simulink model "control_lazo_cerrado_helicoptero"  (R2015a)
settings: Solver=ode45  StartTime=0.0  StopTime=300  RelTol=1e-3
libraries: arduino_io_lib x8
settings Model: CovHtmlReporting=off  Creator=Alumno  LastModifiedBy=Usuario
settings DataIOCC: LimitDataPoints=off  SaveFormat=Dataset
settings HardwareCC: ProdBitPerPointer=64  ProdLargestAtomicFloat=Float  ProdIntDivRoundTo=Zero  ProdEndianess=LittleEndian  ProdHWDeviceType=Specified
settings ModelReferenceCC: PropagateSignalLabelsOutOfModel=on

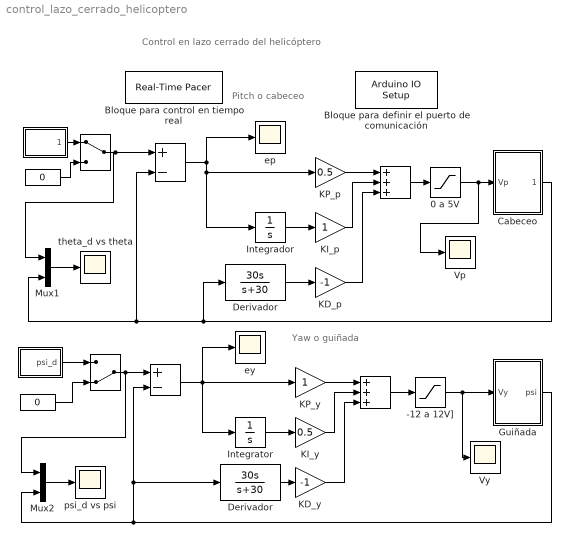
== system control_lazo_cerrado_helicoptero ==
  note: Yaw o guiñada
  note: Pitch o cabeceo
  note: Control en lazo cerrado del helicóptero
  " " : ManualSwitch
  "  " : Sum  Inputs=+-
  "     " : Subsystem
  "       " : Constant  Value=0
  "              " : Sum  Inputs=+++
  "                " : ManualSwitch  CurrentSetting=0
  "                   " : Sum  Inputs=+-
  "                                           " : Constant  Value=0
  "                                                           " : Subsystem
  "                                                            " : Sum  Inputs=+++
  -12 a 12V] : Saturate  UpperLimit=12  LowerLimit=-12
  0 a 5V : Saturate  UpperLimit=5  LowerLimit=0
  Bloque para control en tiempo real : arduino_io_lib/Real-Time Pacer  simTimePerRealTime=1
  Bloque para definir el puerto de comunicación : arduino_io_lib/Arduino IO Setup  Priority=3  arduinoVar=Temporary arduino variable: Arduino1  workspaceVarName=a  comPort=COM11
  Cabeceo : Subsystem
  Derivador : TransferFcn  Numerator=[30 0]  Denominator=[1 30]
  "Derivador " : TransferFcn  Numerator=[30 0]  Denominator=[1 30]
  Guiñada : Subsystem
  "Integrador          " : Integrator
  "Integrator " : Integrator
  KD_p : Gain  Gain=-1
  KD_y : Gain  Gain=-1
  KI_p : Gain
  KI_y : Gain  Gain=0.5
  KP_p : Gain  Gain=0.5
  KP_y : Gain
  Mux1 : Mux  Inputs=2
  Mux2 : Mux  Inputs=2
  Vp : Scope
      settings: YMin=-0.37095  YMax=3.33852  SaveName=ScopeData6
  Vy : Scope
      settings: YMin=-2.30841  YMax=0.77565  SaveName=ScopeData3
  ep : Scope
      settings: YMin=-0.14677  YMax=0.21266  SaveName=ScopeData2
  ey : Scope
      settings: YMin=-19.575  YMax=20.175
  psi_d vs psi : Scope
      settings: YMin=-12.68437  YMax=12.90937
  theta_d vs theta : Scope
      settings: YMin=-12.68437  YMax=12.90937  SaveName=ScopeData2
  wires:
  "                   "/1 -> ey/1, "Integrator "/1, KP_y/1
  Guiñada/1(psi) -> Mux2/2, "                   "/2, "Derivador "/1
  "Integrator "/1 -> KI_y/1
  KP_y/1 -> "                                                            "/1
  KI_y/1 -> "                                                            "/2
  -12 a 12V]/1 -> Vy/1, Guiñada/1(Vy)
  "                                                            "/1 -> -12 a 12V]/1
  "Derivador "/1 -> KD_y/1
  KD_y/1 -> "                                                            "/3
  "  "/1 -> KP_p/1, "Integrador          "/1, ep/1
  Cabeceo/1(theta) -> Mux1/2, "  "/2, Derivador/1
  " "/1 -> Mux1/1, "  "/1
  "Integrador          "/1 -> KI_p/1
  KP_p/1 -> "              "/1
  KI_p/1 -> "              "/2
  0 a 5V/1 -> Cabeceo/1(Vp), Vp/1
  "              "/1 -> 0 a 5V/1
  Derivador/1 -> KD_p/1
  KD_p/1 -> "              "/3
  "     "/1(theta_d) -> " "/1
  "       "/1 -> " "/2
  "                                                           "/1(psi_d) -> "                "/1
  "                                           "/1 -> "                "/2
  Mux1/1 -> theta_d vs theta/1
  "                "/1 -> Mux2/1, "                   "/1
  Mux2/1 -> psi_d vs psi/1

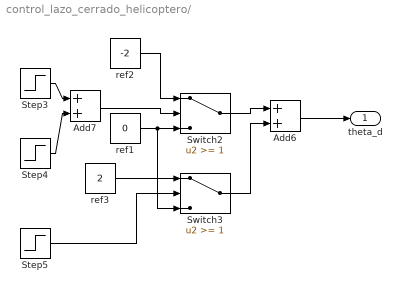
== system control_lazo_cerrado_helicoptero/      ==
  Add6 : Sum
  Add7 : Sum
  Step3 : Step  Time=75  SampleTime=0
  Step4 : Step  Time=150  After=-1  SampleTime=0
  Step5 : Step  Time=150  SampleTime=0
  Switch2 : Switch  Threshold=1
  Switch3 : Switch  Threshold=1
  ref1 : Constant  Value=0
  ref2 : Constant  Value=-2
  ref3 : Constant  Value=2
  theta_d : Outport
  wires:
  ref2/1 -> Switch2/1
  Switch3/1 -> Add6/2
  Step3/1 -> Add7/1
  Step4/1 -> Add7/2
  ref3/1 -> Switch3/1
  Step5/1 -> Switch3/2
  ref1/1 -> Switch3/3, Switch2/3
  Add7/1 -> Switch2/2
  Switch2/1 -> Add6/1
  Add6/1 -> theta_d/1

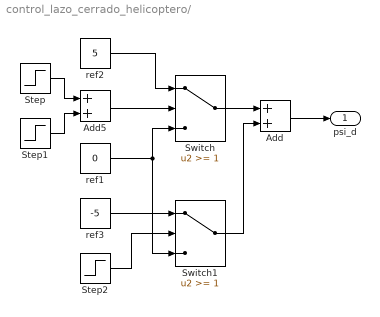
== system control_lazo_cerrado_helicoptero/                                                            ==
  Add : Sum
  Add5 : Sum
  Step : Step  Time=100  SampleTime=0
  Step1 : Step  Time=200  After=-1  SampleTime=0
  Step2 : Step  Time=200  SampleTime=0
  Switch : Switch  Threshold=1
  Switch1 : Switch  Threshold=1
  ref1 : Constant  Value=0
  ref2 : Constant  Value=5
  ref3 : Constant  Value=-5
  psi_d : Outport
  wires:
  ref1/1 -> Switch/3, Switch1/3
  ref2/1 -> Switch/1
  Switch/1 -> Add/1
  Switch1/1 -> Add/2
  Step/1 -> Add5/1
  Step1/1 -> Add5/2
  Add5/1 -> Switch/2
  ref3/1 -> Switch1/1
  Step2/1 -> Switch1/2
  Add/1 -> psi_d/1

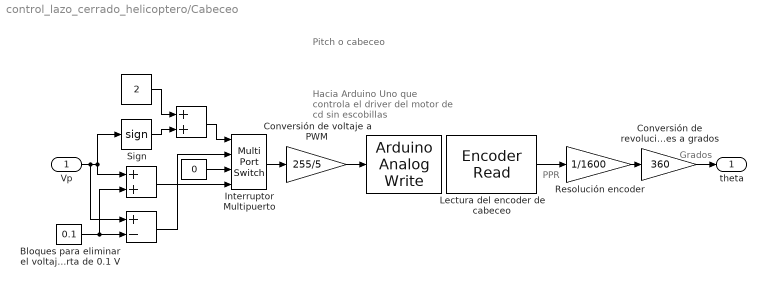
== system control_lazo_cerrado_helicoptero/Cabeceo ==
  note: Pitch o cabeceo
  note: PPR
  note: Grados
  note: Hacia Arduino Uno que
      | controla el driver del motor
      | de cd sin escobillas
  Vp : Inport
  " " : Sum
  "  " : Constant  Value=2
  "        " : Sum
  "                       " : Constant  Value=0
  "                                             " : Sum  Inputs=+-
  "                                                                           " : arduino_io_lib/Arduino Analog Write  arduinoVar=Temporary arduino variable: Arduino1  arduinoPin=7  T=0.02
  "                                   Bloques para eliminar el voltaje de zona muerta de 0.1 V" : Constant  Value=0.1
  Conversión de revoluciones a grados : Gain  Gain=360
  Conversión de voltaje a PWM : Gain  Gain=255/5
  "Interruptor Multipuerto " : MultiPortSwitch
  Lectura del encoder de cabeceo : arduino_io_lib/Encoder Read  arduinoVar=Temporary arduino variable: Arduino1  encNum=1  pinA=18  pinB=19  DbDl=0  T=0.02
  Resolución encoder : Gain  Gain=1/1600
  Sign : Signum  ZeroCross=off
  theta : Outport
  wires:
  Resolución encoder/1 -> Conversión de revoluciones a grados/1
  Conversión de revoluciones a grados/1 -> theta/1
  Lectura del encoder de cabeceo/1 -> Resolución encoder/1
  "                                   Bloques para eliminar el voltaje de zona muerta de 0.1 V"/1 -> " "/2, "                                             "/2
  "        "/1 -> "Interruptor Multipuerto "/1
  "                       "/1 -> "Interruptor Multipuerto "/3
  "  "/1 -> "        "/1
  Sign/1 -> "        "/2
  Vp/1 -> Sign/1, " "/1, "                                             "/1
  " "/1 -> "Interruptor Multipuerto "/4
  "                                             "/1 -> "Interruptor Multipuerto "/2
  "Interruptor Multipuerto "/1 -> Conversión de voltaje a PWM/1
  Conversión de voltaje a PWM/1 -> "                                                                           "/1

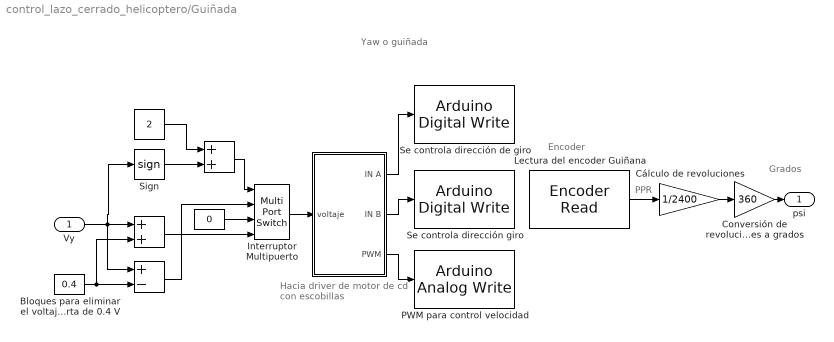
== system control_lazo_cerrado_helicoptero/Guiñada ==
  note: Encoder
  note: Yaw o guiñada
  note: Hacia driver de motor
      | de cd con escobillas
  note: PPR
  note: Grados
  Vy : Inport
  " " : Subsystem
  "  " : Constant  Value=2
  "   " : Sum
  "    " : Sum
  "        " : Sum  Inputs=+-
  "            " : Constant  Value=0
  "                                       Bloques para eliminar el voltaje de zona muerta de 0.4 V" : Constant  Value=0.4
  Conversión de revoluciones a grados : Gain  Gain=360
  Cálculo de revoluciones : Gain  Gain=1/2400
  Interruptor Multipuerto : MultiPortSwitch
  Lectura del encoder Guiñana : arduino_io_lib/Encoder Read  arduinoVar=Temporary arduino variable: Arduino1  encNum=2  pinA=3  pinB=2  DbDl=0  T=0.02
  "PWM para control velocidad " : arduino_io_lib/Arduino Analog Write  arduinoVar=Temporary arduino variable: Arduino1  arduinoPin=10  T=0.02
  "Se controla dirección de giro " : arduino_io_lib/Arduino Digital Write  arduinoVar=Temporary arduino variable: Arduino1  arduinoPin=4  T=0.02
  Se controla dirección giro : arduino_io_lib/Arduino Digital Write  arduinoVar=Temporary arduino variable: Arduino1  arduinoPin=5  T=0.02
  Sign : Signum  ZeroCross=off
  psi : Outport
  wires:
  " "/2(IN B) -> Se controla dirección giro/1
  "                                       Bloques para eliminar el voltaje de zona muerta de 0.4 V"/1 -> "        "/2, "    "/2
  "   "/1 -> Interruptor Multipuerto/1
  " "/1(IN A) -> "Se controla dirección de giro "/1
  "            "/1 -> Interruptor Multipuerto/3
  "  "/1 -> "   "/1
  Sign/1 -> "   "/2
  Interruptor Multipuerto/1 -> " "/1(voltaje)
  Vy/1 -> Sign/1, "        "/1, "    "/1
  "    "/1 -> Interruptor Multipuerto/4
  "        "/1 -> Interruptor Multipuerto/2
  " "/3(PWM) -> "PWM para control velocidad "/1
  Lectura del encoder Guiñana/1 -> Cálculo de revoluciones/1
  Conversión de revoluciones a grados/1 -> psi/1
  Cálculo de revoluciones/1 -> Conversión de revoluciones a grados/1

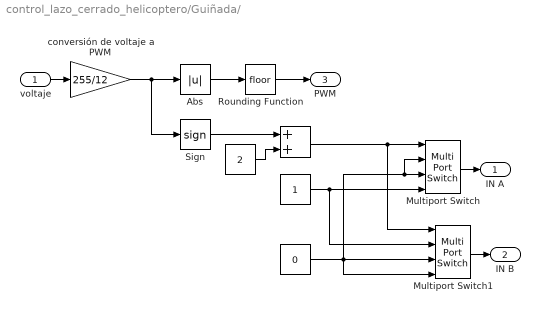
== system control_lazo_cerrado_helicoptero/Guiñada/  ==
  voltaje : Inport
  " " : Constant  Value=2
  "  " : Sum
  "     " : Constant
  "                         " : Constant  Value=0
  Abs : Abs
  Multiport Switch : MultiPortSwitch
  Multiport Switch1 : MultiPortSwitch
  Rounding Function : Rounding
  Sign : Signum
  conversión de voltaje a PWM : Gain  Gain=255/12
  IN A : Outport
  IN B : Outport  Port=2
  PWM : Outport  Port=3
  wires:
  conversión de voltaje a PWM/1 -> Sign/1, Abs/1
  Abs/1 -> Rounding Function/1
  voltaje/1 -> conversión de voltaje a PWM/1
  Sign/1 -> "  "/1
  " "/1 -> "  "/2
  "                         "/1 -> Multiport Switch1/3, Multiport Switch/2, Multiport Switch/3, Multiport Switch1/4
  Multiport Switch/1 -> IN A/1
  Multiport Switch1/1 -> IN B/1
  Rounding Function/1 -> PWM/1
  "  "/1 -> Multiport Switch1/1, Multiport Switch/1
  "     "/1 -> Multiport Switch1/2, Multiport Switch/4
